simulink model "assignment_pil"  (Simulink 9.2)
settings: Solver=FixedStepAuto  StartTime=0.0  StopTime=6.0522e+03  RelTol=1e-3  EnableMultiTasking=on
values from neighbouring files (symbols this model uses):
  a = (r_a + r_p)/2    (= 7178)    [main.m]
  A_BN_0 = quatToAtt(q_0)    [main.m]
  A_epsilon = [cos(psi)*cos(tetha),  cos(psi)*sin(tetha)*sin(phi)+sin(psi)*cos(phi), -cos(psi)*sin(tetha)*cos(phi)+sin(psi)*sin(phi) ... (first row only)    [main.m]
  A_i = [A_i_1, A_i_2, A_i_3]    [main.m]
  a_m = 6371.2    [main.m]
  C_d = 2.2    [main.m]
  dim = [w, l, h]    [main.m]
  i = 60    [main.m]
  I = [I_1,   0,  0 ... (first row only)    [main.m]
  I_inv = inv(I)    [main.m]
  k_bdot = -((4*pi)/((2*pi*sqrt(a^3/mu))) * (1 + sin(deg2rad(48.5))) * min([I_1,I_2,I_3]))*100000    [main.m]
  k_d = -0.07    [main.m]
  k_p = -0.0003    [main.m]
  m_max = 1.2    [main.m]
  max_momentum = 11.076    [main.m]
  max_torque = 0.635    [main.m]
  mu = 398600    [main.m]
  nadir_vector = [1; 0; 0]    [main.m]
  OMG = 0    [main.m]
  omg = 0    [main.m]
  phi_0 = 0    [main.m]
  psi_0 = 0    [main.m]
  q_0 = [0;0;0;1]    [main.m]
  R_e = 6.378e+03    (= 6378)    [main.m]
  rho_d = 0.1    [main.m]
  rho_s = 0.5    [main.m]
  sigma_e = 4.84814e-6    (= 4.84814e-06)    [main.m]
  theta = 0    [main.m]
  theta_0 = 0    [main.m]
  w_0 = [w1_0,w2_0,w3_0]    [main.m]
  w_e = [0 0 0.00007291]    [main.m]
undefined symbols (not defined in the file or in its folder): DiscIntNeverNeededParam, gm, gn, gsvi, gvali, hm, hn, hsvi, hvali, Q_C
libraries: sharedutil x4, sharedtransform x2, aerolibconvert2 x2, simulink x2, vrlib x1
(part 2 of 2)

== matlab function Disturbance Torques/Solar Radiation Pressure Torque Calculator/Subsystem/sunPosition ==
  data: JD input double; S_i output double; r_LVLH input double; S_eartSun output double
function [S_i, S_eartSun]  = sunPosition(JD,r_LVLH)

% Formulas taken from  Fundamentals of Spacecraft
% Attitude Determination and Control pag. 421 

% Number of centuries
T_UT1 = (JD - 2451545.0)/36525;

% Mean longitude of the Sun
phi_sun = 280.460 + 36000.771*T_UT1;

% phi_sun must be in the range 0 - 360 degrees
if (phi_sun >= 360)
    phi_sun = phi_sun - fix(phi_sun/360)*360;
elseif (phi_sun < 0)
    phi_sun = phi_sun - (fix(phi_sun/360) - 1)*360;
end

% Mean anomaly of the Sun
M_sun = 357.5277233 + 35999.05034*T_UT1;

% M_sun must be in the range 0 - 360 degrees
if (M_sun >= 360)
    M_sun = M_sun - fix(M_sun/360)*360;
elseif (M_sun < 0)
    M_sun = M_sun - (fix(M_sun/360) - 1)*360;
end

% Longitude of the ecliptic, in degrees
phi_ecliptic = phi_sun + 1.914666471*sind(M_sun) + 0.019994643*sind(2*M_sun);

% Obliquity of the ecliptic, in degrees
epsilon = 23.439291 - 0.0130042*T_UT1;

% This is the direction from the Earth To the Sun
S_eartSun = [cosd(phi_ecliptic);
             cosd(epsilon)*sind(phi_ecliptic);
             sind(epsilon)*sind(phi_ecliptic)];

% Distance between the Earth and the Sun, in AU  
r_earthSun_mod = 1.000140612 - 0.016708617*cosd(M_sun) - 0.000139589*cosd(2*M_sun);
r_earthSun = r_earthSun_mod*S_eartSun;

% We need r_LVLH in AU
r_LVLH = r_LVLH*6.68459e-9;

% Compute the distance between the S/C and the Sun
r_satSun = r_earthSun - r_LVLH;

% Compute S_i
S_i = r_satSun/norm(r_satSun);

== matlab function Disturbance Torques/Magnetic Field Torque Calculator/Complete Model/Subsystem/MATLAB Function2 ==
  data: jd input double; date output double
function date = jd2date(jd)
%JD2DATE Gregorian calendar date from Julian day number.
%
% DATE = JD2DATE(JD) returns the Gregorian calendar date (year, month, day,
% hour, minute, and second) corresponding to the Julian day number JD.
%
% Note: jd must be a non-negative real. This means that the function is
%       valid for the whole range of dates since 12:00 noon 24 November
%       -4713, Gregorian calendar. (This bound is due to the function
%       FRACDAY2HMS that does not work for negative inputs)
%
% INPUT
%   jd          Date in Julian Day. The JD (Julian day) count is from 0 at
%               12:00 noon, 1 January -4712 (4713 BC), Julian proleptic
%               calendar. The corresponding date in Gregorian calendar is
%               12:00 noon, 24 November -4713. It must be a non-negative
%               real.
%
% OUTPUT
%	date        Date in the Gregorian calendar, as a 6-element vector
%               [year, month, day, hour, minute, second]. For dates before
%               1582, the resulting date components are valid only in the
%               Gregorian proleptic calendar. This is based on the
%               Gregorian calendar but extended to cover dates before its
%               introduction.
%
% REFERENCES
%   Formula from http://en.wikipedia.org/wiki/Julian_day
%   (last visited 16/02/2008)
%   Compared to http://pdc.ro.nu/mjd.cgi for a few dates, the same results
%   were found
%
% See also DATE2JD.
%
% FUNCTIONS CALLED
%   FRACDAY2HMS
%
% - Nicolas Croisard - 16/02/2008
% - Revised by Matteo Ceriotti - 21/02/2008 - Validated with:
%   - Fliegel, Van Flandern "A machine Algorithm for Processing Calendar
%     Dates", Communications of the ACM, 1968. Also on Wertz, "Space
%     Mission Analysis and Design".
%   - A revised version of the algorithm on Vallado, "Fundamentals of
%     Astrodynamics and Applications", third edition, for dates from year
%     1900 to year 2100.
%

% Adding 0.5 to JD and taking FLOOR ensures that the date is correct.
j = floor(jd+0.5) + 32044;
g = floor(j/146097);
dg = mod(j,146097);
c = floor((floor(dg/36524)+1) * 3/4);
dc = dg - c*36524;
b = floor(dc/1461);
db = mod(dc,1461);
a = floor((floor(db/365)+1) * 3/4);
da = db - a*365;
y = g*400 + c*100 + b*4 + a;
m = floor((da*5 + 308)/153) - 2;
d = da - floor((m+4)*153/5) + 122;

% Year, Month and Day
Y = y-4800 + floor((m+2)/12);
M = mod((m+2),12) + 1;
D = floor(d+1);

% Hour, Minute and Second
[hrs, mn, sec] = fracday2hms(mod(jd+0.5,floor(jd+0.5)));

% Prepare output
date = [Y, M, D, hrs, mn, sec];

== matlab function On-Board Computer/Kinematics/ /MATLAB Function ==
  data: w_ln_cross input double; w_ln output double
function w_ln = w_component_extractor(w_ln_cross)

w_1 = w_ln_cross(3,2);
w_2 = w_ln_cross(1,3);
w_3 = w_ln_cross(2,1);

w_ln = [w_1, w_2, w_3]';
end

== matlab function Disturbance Torques/Solar Radiation Pressure Torque Calculator/MATLAB Function ==
  data: r input double; R_e input double; S_b input double; S_earthSun input double; srp_torque output double; A_i input double; dim input double; rho_d input double; rho_s input double
function srp_torque  = srp(r, R_e, S_b, S_earthSun, A_i, dim, rho_d, rho_s)

% Define normal vectors
n_1 = [1 0 0];
n_2 = [0 1 0];
n_3 = [0 0 1];
n_4 = [-1 0 0];
n_5 = [0 -1 0];
n_6 = [0 0 -1];

% Dimensions 
w = dim(1);
l = dim(2);
h = dim(3);

% Sections 
A_i_1 = A_i(1);
A_i_2 = A_i(2);
A_i_3 = A_i(3);
A_i_4 = A_i(1);
A_i_5 = A_i(2);
A_i_6 = A_i(3);

% Distance between the center of pressure and the center of mass
% +0.1*rcg(da aggiungere)
r_1 = [h/2 0.1 0.1];
r_2 = [0.2 l/2 0.2];
r_3 = [0.4 0.4 w/2];
r_4 = [-h/2 0.1 0.1];
r_5 = [0.2 -l/2 0.2];
r_6 = [0.4 0.4 -w/2];

% Values taken from  Fundamentals of Spacecraft
% Attitude Determination and Control pag. 421
solar_flux = 1362;        % W/m^2
c = 299792458;            % m/s
P = solar_flux/c;         % Pa

S_b = S_b';

% Compute SRP on all the surface only if we are not shadowed by the Earth
if dot(r,S_earthSun) < -sqrt((norm(r))^2 - R_e^2)
    srp_torque = [0 0 0]';
else    
    % Compute torque due to the solar radiation pressure only exposed faces.
    % If dot(S_b,n_i)) => 1 then the face is exposed othewise no.
    if dot(S_b,n_1) >= 0
        F_srp_1 = P*A_i_1*dot(S_b,n_1) * ((1-rho_s)*S_b + (2*rho_s*dot(S_b,n_1)+2/3*rho_d)*n_1);
        T_srp_1 = cross(r_1,F_srp_1);
    else
        T_srp_1 = [0 0 0];
    end
    
    if dot(S_b,n_2) >= 0
        F_srp_2 = P*A_i_2*dot(S_b,n_2) * ((1-rho_s)*S_b + (2*rho_s*dot(S_b,n_2)+2/3*rho_d)*n_2);
        T_srp_2 = cross(r_2,F_srp_2);
    else
        T_srp_2 = [0 0 0];
    end
    
    if dot(S_b,n_3) >= 0
        F_srp_3 = P*A_i_3*dot(S_b,n_3) * ((1-rho_s)*S_b + (2*rho_s*dot(S_b,n_3)+2/3*rho_d)*n_3);
        T_srp_3 = cross(r_3,F_srp_3);
    else
        T_srp_3 = [0 0 0];
    end
    
    if dot(S_b,n_4) >= 0
        F_srp_4 = P*A_i_4*dot(S_b,n_4) * ((1-rho_s)*S_b + (2*rho_s*dot(S_b,n_4)+2/3*rho_d)*n_4);
        T_srp_4 = cross(r_4,F_srp_4);
    else
        T_srp_4 = [0 0 0];
    end
    
    if dot(S_b,n_5) >= 0
        F_srp_5 = P*A_i_5*dot(S_b,n_5) * ((1-rho_s)*S_b + (2*rho_s*dot(S_b,n_5)+2/3*rho_d)*n_5);
        T_srp_5 = cross(r_5,F_srp_5);
    else
        T_srp_5 = [0 0 0];
    end
    
    if dot(S_b,n_6) >= 0
        F_srp_6 = P*A_i_6*dot(S_b,n_6) * ((1-rho_s)*S_b + (2*rho_s*dot(S_b,n_6)+2/3*rho_d)*n_6);
        T_srp_6 = cross(r_6,F_srp_6);
    else
        T_srp_6 = [0 0 0];
    end
    % Compute Solar Radiation Pressure on all surfaces
    srp_torque = [T_srp_1 + T_srp_2 + T_srp_3 + T_srp_4 + T_srp_5 + T_srp_5 + T_srp_6]';
end

end

== matlab function Disturbance Torques/Magnetic Field Torque Calculator/Complete Model/MATLAB Function ==
  data: r input double; theta input double; phi input double; IGRF_coefficients input double; B output double; days input double; theta_LST input double; a input double
function B  = magnet(r, theta, phi, IGRF_coefficients, days, theta_LST, a)

% Inputs
%   r       Geocentric radius measured in kilometers
%   theta   Latitude measured in degrees positive from equator
%   phi     Longitude measured in degrees positive from Greenwich
%   days    Date in MJD2000 Format
%   a       Reference radius used in IGRF measured in kilometers
%

% Checks to see if located at either pole to avoid singularities
if (theta>-0.00000001 && theta<0.00000001)
    theta=0.00000001;
elseif(theta<180.00000001 && theta>179.99999999)
    theta=179.99999999;
end

% Store the latitude in a seperate variable so we can use it later for
% frame rotation
lat = theta;

% The angles must be converted from degrees into radians 
theta=(90-theta)*pi/180;
phi = phi*pi/180;

% This section of the code simply reads in the g and h Schmidt
% quasi-normalized coefficients from a mat file
gn = IGRF_coefficients(:,1);
gm = IGRF_coefficients(:,2);
gvali = IGRF_coefficients(:,3);
gsvi = IGRF_coefficients(:,4);
hn = IGRF_coefficients(:,5);
hm = IGRF_coefficients(:,6);
hvali = IGRF_coefficients(:,7);
hsvi = IGRF_coefficients(:,8);

% For some reason Simlink does not allow to compute N as max of gn vector,
% so since those values are fixed, put N=10 directly
% N=max(gn);
N = 10;
g = zeros(N,N+1);
h = zeros(N,N+1);

for x=1:length(gn)
    g(gn(x),gm(x)+1) = gvali(x) + gsvi(x)*days/365;
    h(hn(x),hm(x)+1) = hvali(x) + hsvi(x)*days/365;
end

% Initialize the variables
% Br    B in the radial direction
% Bt    B in the theta direction
% Bp    B in the phi direction
% P     The associated Legendre polynomial evaluated at cos(theta)
%       The nomenclature for the recursive values generally follows
%       the form P10 = P(n-1,m-0)
% dP    The partial derivative of P with respect to theta
Br = 0; Bt = 0; Bp = 0;
P11 = 1; P10 = P11;
dP11 = 0; dP10 = dP11;
P20 = 0; dP20 = 0;

% Compute the magnetic field strenght in local tangential coordinates with
% recursive formulas
for m=0:N
    for n=1:N
        if m<=n
            % Compute the Legendre polynomials and their derivatives
            % recursively
            if n == m
                P2 = sin(theta)*P11;
                dP2 = sin(theta)*dP11 + cos(theta)*P11;
                P11 = P2; P10 = P11; P20 = 0;
                dP11 = dP2; dP10 = dP11; dP20 = 0;
            elseif n == 1
                P2 = cos(theta)*P10;
                dP2 = cos(theta)*dP10 - sin(theta)*P10;
                P20 = P10; P10 = P2;
                dP20 = dP10; dP10 = dP2;
            else
                K = ((n-1)^2-m^2)/((2*n-1)*(2*n-3));
                P2 = cos(theta)*P10 - K*P20;
                dP2 = cos(theta)*dP10 - sin(theta)*P10 - K*dP20;
                P20 = P10; P10 = P2;
                dP20 = dP10; dP10 = dP2;
            end
            
            % Calculate Br, Bt, and Bp
            Br = Br + (a/r)^(n+2)*(n+1)*...
                ((g(n,m+1)*cos(m*phi) + h(n,m+1)*sin(m*phi))*P2);
            Bt = Bt + (a/r)^(n+2)*...
                ((g(n,m+1)*cos(m*phi) + h(n,m+1)*sin(m*phi))*dP2);
            Bp = Bp + (a/r)^(n+2)*...
                (m*(-g(n,m+1)*sin(m*phi) + h(n,m+1)*cos(m*phi))* P2);
        end
    end
end

Bt = -Bt;
Bp = -Bp/sin(theta);

% Convert latitude and LST from degrees to radians
lat = lat*pi/180;
theta_LST = theta_LST*pi/180;

% Convert Br, Bt, Bp from tangential spherical to GCI coordinates
Bx = (Br*cos(lat)+Bt*sin(lat))*cos(theta_LST) - Bp*sin(theta_LST);
By = (Br*cos(lat)+Bt*sin(lat))*sin(theta_LST) + Bp*cos(theta_LST);
Bz = (Br*sin(lat)-Bt*cos(lat));

% Compute the Magnetic Field Vector in Tesla
B = [Bx; By; Bz]*1e-9;

== matlab function Disturbance Torques/Gravity Gradient/MATLAB Function ==
  data: u input double; y output double
function y  = norm3(u)

y = (norm(u))^3;

end

== matlab function Disturbance Torques/Magnetic Field Torque Calculator/Complete Model/fromGCItoECEF/MATLAB Function1 ==
  data: r output double; r_LVLH input double; theta_GMST input double; lat output double; lon output double
function [r, lat, lon] = fromGCItoECEF(r_LVLH, theta_GMST)

% Rotation matrix ECEF-GCI 
A_EL = [cos(theta_GMST), sin(theta_GMST), 0;
       -sin(theta_GMST), cos(theta_GMST), 0;
                  0              0        1];
 
r_e = A_EL*r_LVLH;

% Compute geocentric radius
r = norm(r_e);

% Compute latitude
lat = asin(r_e(3)/r);

% Compute longitude
if r_e(2) > 0
    lon = acos(r_e(1)/r/cos(lat));
else
    lon = 2*pi - acos(r_e(1)/r/cos(lat));
end
  
 if lon > pi
     lon = lon - 2*pi;
 end 

% Output latitude and longitude in degrees
lon = rad2deg(lon);
lat = rad2deg(lat);

== matlab function Disturbance Torques/Magnetic Field Torque Calculator/Complete Model/Subsystem/MATLAB Function ==
  data: JD input double; GMST output double; theta_GMST output double
function [GMST, theta_GMST] = JD2GMST(JD)

% Find the Julian Date of the previous midnight, JD0. Adding 0.5 to 
% JD and taking FLOOR ensures that the date is correct.
JD0 = zeros(size(JD));
JDmin = floor(JD)-.5;
JDmax = floor(JD)+.5;
JD0(JD > JDmin) = JDmin(JD > JDmin);
JD0(JD > JDmax) = JDmax(JD > JDmax);

% Time in hours past previous midnight
H = (JD-JD0)*24;                      

% Compute the number of centuries since J2000
T0 = (JD - 2451545.0)/36525; 

% Compute the GMST in hours, formula adapted from Fundamentals of 
% Spacecraft Attitude Determination and Control pag 34
GMST = 6.6973745583333 + 2400.0513369072223*T0 + 2.586222222e-5*T0^2 - 1.7222e-9 *T0^3 + 1.002737909350795*H;

% Compute GMST in degrees 
theta_GMST = GMST*15;

% theta_GMST must be in the range 0 - 360 degrees
if (theta_GMST >= 360)
    theta_GMST = theta_GMST - fix(theta_GMST/360)*360;
elseif (theta_GMST < 0)
    theta_GMST = theta_GMST - (fix(theta_GMST/360) - 1)*360;
end

== matlab function Disturbance Torques/Magnetic Field Torque Calculator/Complete Model/Subsystem/MATLAB Function1 ==
  data: theta_GMST input double; lon input double; theta_LST output double; date input double
function theta_LST = LST(theta_GMST, lon, date)

% Compute Universal Time in hours
ut = date(4) + date(5)/60 + date(6)/3600;

% Formula taken from Curtis page 261
theta_LST = theta_GMST + 360.98564724*(ut/24) + lon;

% Reduce theta_LST to the range 0 - 360 degrees
theta_LST = theta_LST - 360*fix(theta_LST/360);

== matlab function On-Board Computer/Kinematics/LVLH/Full Orbital Dynamics/Compute R and V of reference orbit/Initial Position/MATLAB Function2 ==
  data: r_0 output double; kep input double; mu input double
function r_0  = kep2car(kep,mu)

% Using kep2car function to find position and velocity at initial condition
[r_0,~]=kep2car(kep,mu);

end

== matlab function Actuators/Reaction Wheels/Reaction Wheels Dynamics /MATLAB Function ==
  data: h_d_dot input double; h_d input double; w_bn input double; u output double
function u   = rotationWheel(h_d_dot, h_d, w_bn)

% Actuators attitude matrix
A = [0 0 0;
     0 0 0;
     0 0 1];
 
% Control torque and momentum in body frame
u = cross((A*h_d),w_bn) - A*h_d_dot;

end

== matlab function On-Board Computer/Kinematics/Quaternions/MATLAB Function ==
  data: w input double; w_cross output double
function w_cross  = assembly_w_cross(w)

w_cross = [0, -w(3), w(2);
           w(3), 0, -w(1);
          -w(2), w(1), 0];

== matlab function On-Board Computer/Kinematics/Quaternions/MATLAB Function1 ==
  data: u input double; y output double
function y = ortonormalize(u)
%#codegen
% Ortonormalize a matrix.
% Reference : Lecture 7, Slide 5 SADC Polimi

y = u.*3/2 - u*u'*(u./2);

y = u;

end

== matlab function On-Board Computer/Kinematics/Quaternions/Quaternions/Quaternion Kinematics ==
  data: q input double size=4; q_dot output double size=4; omega input double size=3
function q_dot = quat_kin(q, omega)

qnorm = sqrt(q(1)^2 + q(2)^2 + q(3)^2 + q(4)^2);
q = q./qnorm;

W = [ q(4) -q(3)  q(2) ;
      q(3)  q(4) -q(1) ;
     -q(2)  q(1)  q(4) ; 
     -q(1) -q(2) -q(3)];

q_dot = 0.5 * W * omega;

== matlab function On-Board Computer/ω norm/MATLAB Function1 ==
  data: u input double; y output double
function y = fcn(u)

y = norm(u);

== matlab function On-Board Computer/Kinematics/LVLH/Full Orbital Dynamics/Compute R and V of reference orbit/Initial Velocity/MATLAB Function1 ==
  data: r_dot_0 output double; kep input double; mu input double
function r_dot_0  = kep2car(kep,mu)

% Using kep2car function to find velocity at initial condition
[~,r_dot_0]=kep2car(kep,mu);

end

== matlab function On-Board Computer/Kinematics/LVLH/Full Orbital Dynamics/Compute R and V of reference orbit/Orbital Dynamics ==
  data: r input double; r_dot_dot output double; mu input double
function r_dot_dot  = orbit_equation(r,mu)

r_dot_dot = -(mu/norm(r)^3)*r;

end

== matlab function On-Board Computer/Kinematics/LVLH/Full Orbital Dynamics/MATLAB Function ==
  data: r input double; A_LN output double; r_dot input double
function A_LN = assembly_A_LN(r,r_dot)
% This M-Function builds an LVLH frame from a position vector and a 
% velocity vector

r = r';
r_dot = r_dot';

o_1 = - r/norm(r);                                      % Points toward the Earth, aligned with S/C - Earth direction (x)
o_3 = - (cross(r,r_dot))/(norm(cross(r,r_dot)));         % Points in the direction of angular momentum vector (z)
o_2 = cross(o_3,o_1);                                   % Points into the direction of the motion (y)

A_LN = [o_1; o_2; o_3];

end
